simulink model "EMPCTower"  (R2021a)
settings: Solver=FixedStepDiscrete  StartTime=0.0  StopTime=120  FixedStep=Parameters.Ts  RelTol=1e-3
values from neighbouring files (symbols this model uses):
  Parameters =     [Parameters.mat]
undefined symbols (not defined in the file or in its folder): DeriveCp, DeriveFT, DriveTrain, EMPCController_Tower, TowerDynamic
settings Model: Creator=zfeng1  LastModifiedBy=zfeng1

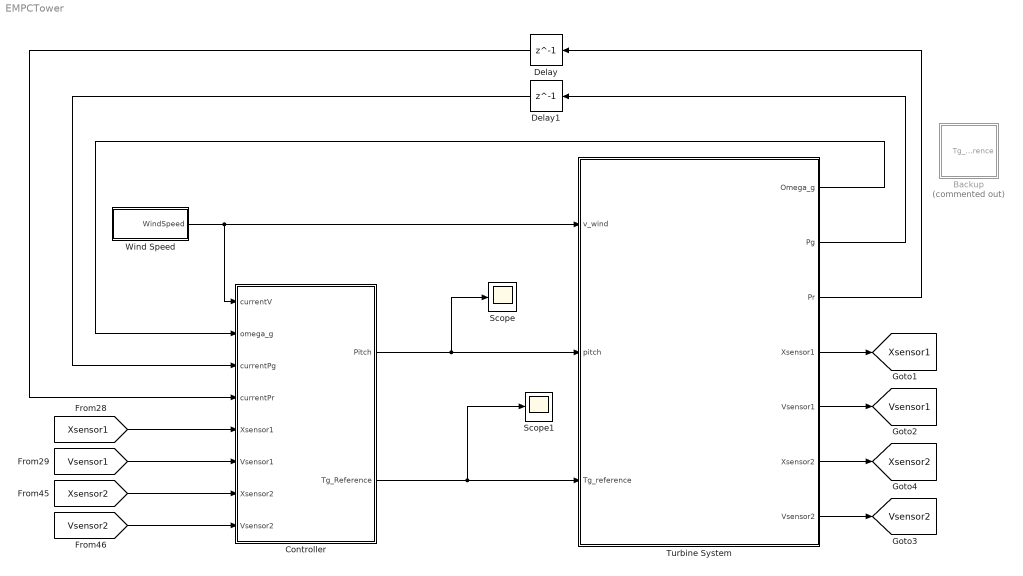
== system EMPCTower ==
  Backup : Subsystem  Commented=on
  Controller : Subsystem
  Delay : Delay  DelayLength=1  InitialCondition=0
  Delay1 : Delay  DelayLength=1  InitialCondition=0
  Scope : Scope
  Scope1 : Scope
  Turbine System : Subsystem
  Wind Speed : Subsystem
  tag scope: Vsensor1=global, Vsensor2=global, Xsensor1=global, Xsensor2=global
  wires:
  [Vsensor1] -> Controller/6(Vsensor1)
  [Vsensor2] -> Controller/8(Vsensor2)
  [Xsensor2] -> Controller/7(Xsensor2)
  [Xsensor1] -> Controller/5(Xsensor1)
  Wind Speed/1(WindSpeed) -> Controller/1(currentV), Turbine System/1(v_wind)
  Controller/1(Pitch) -> Scope/1, Turbine System/2(pitch)
  Controller/2(Tg_Reference) -> Scope1/1, Turbine System/3(Tg_reference)
  Turbine System/4(Xsensor1) -> [Xsensor1]
  Turbine System/5(Vsensor1) -> [Vsensor1]
  Turbine System/6(Xsensor2) -> [Xsensor2]
  Turbine System/7(Vsensor2) -> [Vsensor2]
  Turbine System/3(Pr) -> Delay/1
  Delay/1 -> Controller/4(currentPr)
  Turbine System/2(Pg) -> Delay1/1
  Delay1/1 -> Controller/3(currentPg)
  Turbine System/1(Omega_g) -> Controller/2(omega_g)

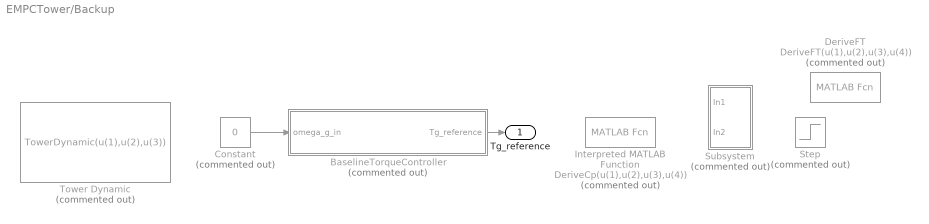
== system EMPCTower/Backup ==
  BaselineTorqueController : MATLAB Function  Commented=on  TreatAsAtomicUnit=on
  Constant : Constant  Commented=on  Value=0
  DeriveFT : MATLABFcn  Commented=on  MATLABFcn=DeriveFT(u(1),u(2),u(3),u(4))
  Interpreted MATLAB Function : MATLABFcn  Commented=on  MATLABFcn=DeriveCp(u(1),u(2),u(3),u(4))
  Step : Step  Commented=on  Time=200  Before=11  After=12  SampleTime=0
  Subsystem : Subsystem  Commented=on
  Tower Dynamic : MATLABFcn  Commented=on  MATLABFcn=TowerDynamic(u(1),u(2),u(3))
  Tg_reference : Outport
  wires:
  Constant/1 -> BaselineTorqueController/1(omega_g_in)
  BaselineTorqueController/1(Tg_reference) -> Tg_reference/1

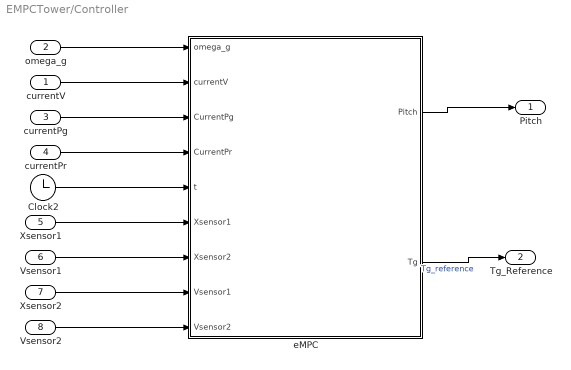
== system EMPCTower/Controller ==
  currentV : Inport
  omega_g : Inport  Port=2
  currentPg : Inport  Port=3
  currentPr : Inport  Port=4
  Xsensor1 : Inport  Port=5
  Vsensor1 : Inport  Port=6
  Xsensor2 : Inport  Port=7
  Vsensor2 : Inport  Port=8
  Clock2 : Clock
  eMPC : Subsystem
  Pitch : Outport
  Tg_Reference : Outport  Port=2
  wires:
  omega_g/1 -> eMPC/1(omega_g)
  currentV/1 -> eMPC/2(currentV)
  Clock2/1 -> eMPC/5(t)
  eMPC/1(Pitch) -> Pitch/1
  Xsensor1/1 -> eMPC/6(Xsensor1)
  Vsensor1/1 -> eMPC/7(Xsensor2)
  Xsensor2/1 -> eMPC/8(Vsensor1)
  Vsensor2/1 -> eMPC/9(Vsensor2)
  eMPC/2(Tg) -> Tg_Reference/1  "Tg_reference"
  currentPg/1 -> eMPC/3(CurrentPg)
  currentPr/1 -> eMPC/4(CurrentPr)

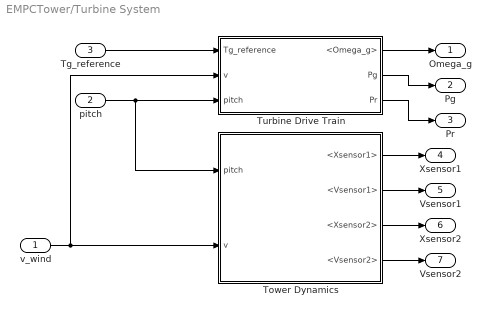
== system EMPCTower/Turbine System ==
  v_wind : Inport
  pitch : Inport  Port=2
  Tg_reference : Inport  Port=3
  Tower Dynamics : Subsystem
  Turbine Drive Train : Subsystem
  Omega_g : Outport
  Pg : Outport  Port=2
  Pr : Outport  Port=3
  Xsensor1 : Outport  Port=4
  Vsensor1 : Outport  Port=5
  Xsensor2 : Outport  Port=6
  Vsensor2 : Outport  Port=7
  wires:
  pitch/1 -> Turbine Drive Train/3(pitch), Tower Dynamics/1(pitch)
  v_wind/1 -> Turbine Drive Train/2(v), Tower Dynamics/2(v)
  Tg_reference/1 -> Turbine Drive Train/1(Tg_reference)
  Turbine Drive Train/1(<Omega_g>) -> Omega_g/1
  Tower Dynamics/1(<Xsensor1>) -> Xsensor1/1
  Tower Dynamics/2(<Vsensor1>) -> Vsensor1/1
  Tower Dynamics/3(<Xsensor2>) -> Xsensor2/1
  Tower Dynamics/4(<Vsensor2>) -> Vsensor2/1
  Turbine Drive Train/3(Pr) -> Pr/1
  Turbine Drive Train/2(Pg) -> Pg/1

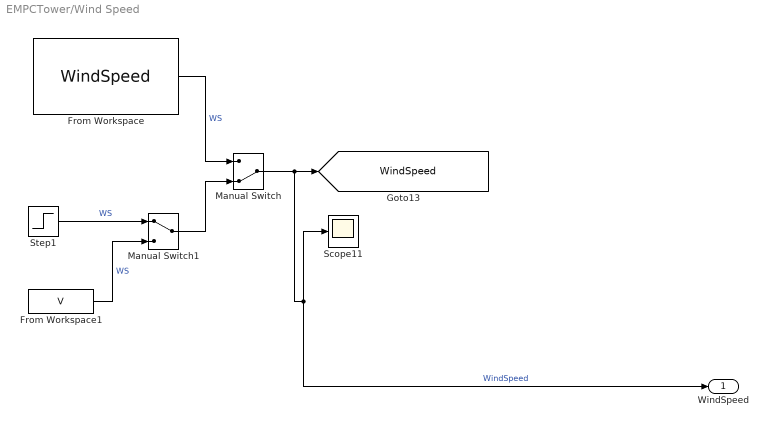
== system EMPCTower/Wind Speed ==
  From Workspace : FromWorkspace  VariableName=WindSpeed  SampleTime=Parameters.Ts
  From Workspace1 : FromWorkspace  VariableName=V
  Manual Switch : ManualSwitch  CurrentSetting=0
  Manual Switch1 : ManualSwitch
  Scope11 : Scope
  Step1 : Step  Time=0  Before=5  After=6  SampleTime=0
  WindSpeed : Outport
  tag scope: WindSpeed=global
  wires:
  Manual Switch1/1 -> Manual Switch/2
  Step1/1 -> Manual Switch1/1  "WS"
  Manual Switch/1 -> WindSpeed/1, Scope11/1, [WindSpeed]  "WindSpeed"
  From Workspace/1 -> Manual Switch/1  "WS"
  From Workspace1/1 -> Manual Switch1/2  "WS"

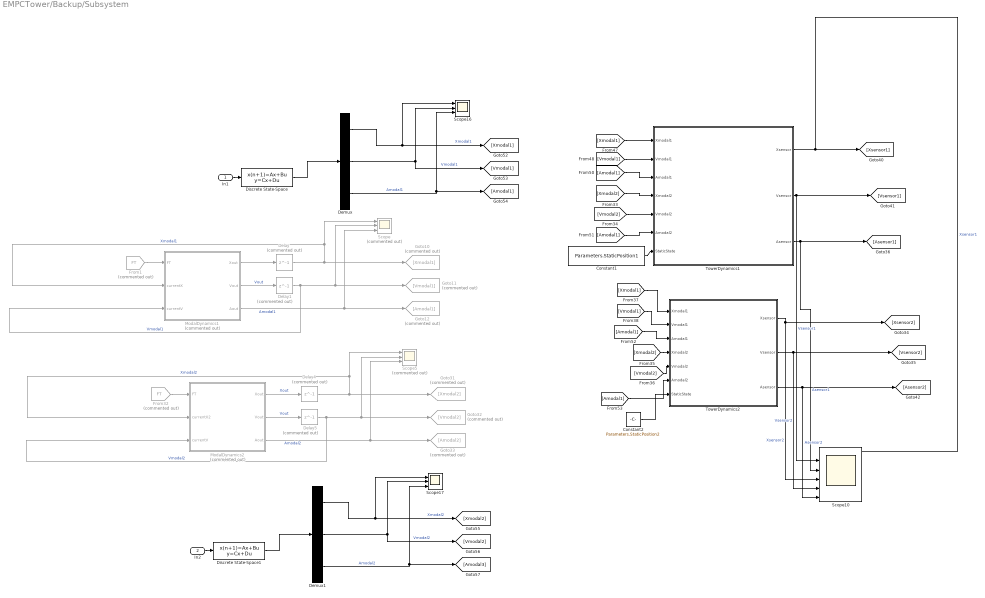
== system EMPCTower/Backup/Subsystem ==
  In1 : Inport
  In2 : Inport  Port=2
  Constant1 : Constant  Value=Parameters.StaticPosition1
  Constant2 : Constant  Value=Parameters.StaticPosition2
  Delay{,1,4..5} (4 alike) : Delay  Commented=on  DelayLength=1  InitialCondition=0  SampleTime=Parameters.Ts
  Demux : Demux  Outputs=3
  Demux1 : Demux  Outputs=3
  Discrete State-Space : DiscreteStateSpace  A=Parameters.sys_tower_fa_d.Am1  B=Parameters.sys_tower_fa_d.Bm1  C=Parameters.sys_tower_fa_d.Cm1  D=Parameters.sys_tower_fa_d.Dm1  SampleTime=-1
  Discrete State-Space1 : DiscreteStateSpace  A=Parameters.sys_tower_fa_d.Am2  B=Parameters.sys_tower_fa_d.Bm2  C=Parameters.sys_tower_fa_d.Cm2  D=Parameters.sys_tower_fa_d.Dm2  SampleTime=-1
  From1 : From  Commented=on  GotoTag=FT
  From32 : From  Commented=on  GotoTag=FT
  Goto10 : Goto  Commented=on  GotoTag=Xmodal1
  Goto11 : Goto  Commented=on  GotoTag=Vmodal1
  Goto12 : Goto  Commented=on  GotoTag=Amodal1
  Goto31 : Goto  Commented=on  GotoTag=Xmodal2
  Goto32 : Goto  Commented=on  GotoTag=Vmodal2
  Goto33 : Goto  Commented=on  GotoTag=Amodal2
  ModalDynamics1 : MATLAB Function  Commented=on  TreatAsAtomicUnit=on
  ModalDynamics2 : MATLAB Function  Commented=on  TreatAsAtomicUnit=on
  Scope : Scope  Commented=on  NumInputPorts=3
  Scope10 : Scope  NumInputPorts=6
  Scope16 : Scope  NumInputPorts=3
  Scope17 : Scope  NumInputPorts=3
  Scope5 : Scope  Commented=on  NumInputPorts=3
  TowerDynamics1 : MATLAB Function  TreatAsAtomicUnit=on
  TowerDynamics2 : MATLAB Function  TreatAsAtomicUnit=on
  wires:
  TowerDynamics1/2(Vsensor) -> [Vsensor1], Scope10/2  "Vsensor1"
  Demux/3 -> Scope16/3, [Amodal1]  "Amodal1"
  In1/1 -> Discrete State-Space/1
  ModalDynamics1/3(Aout) -> Scope/3, Goto12/1  "Amodal1"
  Delay4/1 -> ModalDynamics2/2(currentX2), Scope5/1, Goto31/1  "Xmodal2"
  In2/1 -> Discrete State-Space1/1
  Demux/2 -> Scope16/2, [Vmodal1]  "Vmodal1"
  Demux1/2 -> Scope17/2, [Vmodal2]  "Vmodal2"
  Discrete State-Space1/1 -> Demux1/1
  From1/1 -> ModalDynamics1/1(FT)
  Demux1/3 -> Scope17/3, [Amodal3]  "Amodal2"
  Demux/1 -> Scope16/1, [Xmodal1]  "Xmodal1"
  Discrete State-Space/1 -> Demux/1
  Constant1/1 -> TowerDynamics1/7(StaticState)
  [Vmodal1] -> TowerDynamics1/2(Vmodal1)
  ModalDynamics1/1(Xout) -> Delay/1
  TowerDynamics1/1(Xsensor) -> [Xsensor1], Scope10/1  "Xsensor1"
  [Amodal1] -> TowerDynamics2/6(Amodal2)
  [Amodal1] -> TowerDynamics1/6(Amodal2)
  ModalDynamics1/2(Vout) -> Delay1/1  "Vout"
  Delay/1 -> ModalDynamics1/2(currentX), Scope/1, Goto10/1  "Xmodal1"
  ModalDynamics2/3(Aout) -> Scope5/3, Goto33/1  "Amodal2"
  [Amodal1] -> TowerDynamics2/3(Amodal1)
  TowerDynamics2/3(Asensor) -> Scope10/6, [Asensor2]  "Asensor2"
  Constant2/1 -> TowerDynamics2/7(StaticState)
  Delay1/1 -> ModalDynamics1/3(currentV), Goto11/1, Scope/2  "Vmodal1"
  TowerDynamics1/3(Asensor) -> Scope10/3, [Asensor1]  "Asensor1"
  ModalDynamics2/2(Vout) -> Delay5/1  "Vout"
  [Xmodal2] -> TowerDynamics2/4(Xmodal2)
  [Vmodal2] -> TowerDynamics1/5(Vmodal2)
  [Xmodal1] -> TowerDynamics2/1(Xmodal1)
  ModalDynamics2/1(Xout) -> Delay4/1  "Xout"
  [Xmodal1] -> TowerDynamics1/1(Xmodal1)
  [Xmodal2] -> TowerDynamics1/4(Xmodal2)
  TowerDynamics2/2(Vsensor) -> Scope10/5, [Vsensor2]  "Vsensor2"
  From32/1 -> ModalDynamics2/1(FT)
  [Vmodal2] -> TowerDynamics2/5(Vmodal2)
  [Amodal1] -> TowerDynamics1/3(Amodal1)
  [Vmodal1] -> TowerDynamics2/2(Vmodal1)
  TowerDynamics2/1(Xsensor) -> Scope10/4, [Xsensor2]  "Xsensor2"
  Delay5/1 -> ModalDynamics2/3(currentV), Goto32/1, Scope5/2  "Vmodal2"
  Demux1/1 -> Scope17/1, [Xmodal2]  "Xmodal2"

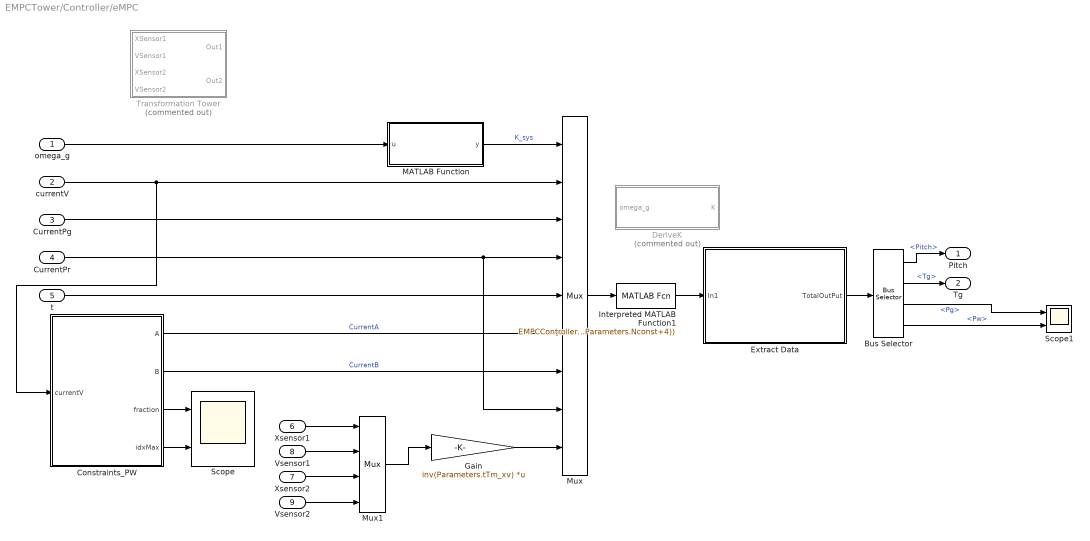
== system EMPCTower/Controller/eMPC ==
  omega_g : Inport
  currentV : Inport  Port=2
  CurrentPg : Inport  Port=3
  CurrentPr : Inport  Port=4
  t : Inport  Port=5
  Xsensor1 : Inport  Port=6
  Xsensor2 : Inport  Port=7
  Vsensor1 : Inport  Port=8
  Vsensor2 : Inport  Port=9
  Bus Selector : BusSelector  OutputSignals=Pitch,Tg,Pg,Pw
  Constraints_PW : MATLAB Function  TreatAsAtomicUnit=on  SystemSampleTime=Parameters.Ts
  DeriveK : MATLAB Function  Commented=on  TreatAsAtomicUnit=on  SystemSampleTime=Parameters.DT
  Extract Data : Subsystem
  Gain : Gain  Gain=inv(Parameters.tTm_xv)  Multiplication=Matrix(K*u) (u vector)
  Interpreted MATLAB Function1 : MATLABFcn  MATLABFcn=EMPCController_Tower(u(1),u(2),u(3),u(4),u(5),u(6:1:6+Parameters.Nconst-1),u(6+Parameters.Nconst:1:6+2*Parameters.Nconst-1),u(6+2*Parameters.Nconst),u(6+2*Parameters.Nconst+1:6+2*Parameters.Nconst+2),u(6+2*Parameters.Nconst+3:6+2*Parameters.Nconst+4))
  MATLAB Function : MATLAB Function  TreatAsAtomicUnit=on
  Mux : Mux  Inputs=9
  Mux1 : Mux
  Scope : Scope  NumInputPorts=2
  Scope1 : Scope  NumInputPorts=2
  Transformation Tower : Subsystem  Commented=on
  Pitch : Outport
  Tg : Outport  Port=2
  wires:
  Constraints_PW/1(A) -> Mux/6  "CurrentA"
  currentV/1 -> Mux/2, Constraints_PW/1(currentV)
  Mux/1 -> Interpreted MATLAB Function1/1
  MATLAB Function/1(y) -> Mux/1  "K_sys"
  Constraints_PW/2(B) -> Mux/7  "CurrentB"
  omega_g/1 -> MATLAB Function/1(u)
  t/1 -> Mux/5
  Constraints_PW/3(fraction) -> Scope/1
  Constraints_PW/4(idxMax) -> Scope/2
  Interpreted MATLAB Function1/1 -> Extract Data/1(In1)
  Xsensor1/1 -> Mux1/1
  Vsensor1/1 -> Mux1/2
  Xsensor2/1 -> Mux1/3
  Vsensor2/1 -> Mux1/4
  Mux1/1 -> Gain/1
  Extract Data/1(TotalOutPut) -> Bus Selector/1
  Bus Selector/1 -> Pitch/1  "<Pitch>"
  Bus Selector/2 -> Tg/1  "<Tg>"
  Bus Selector/3 -> Scope1/1  "<Pg>"
  Bus Selector/4 -> Scope1/2  "<Pw>"
  Gain/1 -> Mux/9
  CurrentPg/1 -> Mux/3
  CurrentPr/1 -> Mux/8, Mux/4

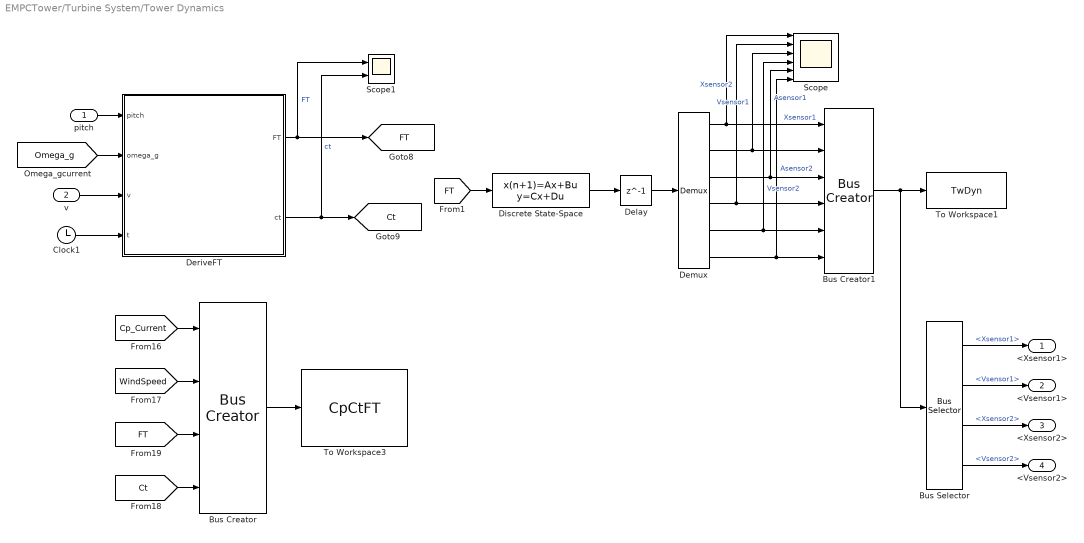
== system EMPCTower/Turbine System/Tower Dynamics ==
  pitch : Inport
  v : Inport  Port=2
  " DeriveFT" : MATLAB Function  TreatAsAtomicUnit=on
  Bus Creator : BusCreator  Inputs=4
  Bus Creator1 : BusCreator  Inputs=6
  Bus Selector : BusSelector  OutputSignals=Xsensor1,Vsensor1,Xsensor2,Vsensor2
  Clock1 : Clock
  Delay : Delay  DelayLength=1  InitialCondition=0
  Demux : Demux  Outputs=6
  Discrete State-Space : DiscreteStateSpace  A=Parameters.sys_tower_fa_d.A  B=Parameters.sys_tower_fa_d.B  C=Parameters.sys_tower_fa_d.C  D=Parameters.sys_tower_fa_d.D  SampleTime=Parameters.Ts
  Scope : Scope  NumInputPorts=6
  Scope1 : Scope  NumInputPorts=2
  To Workspace1 : ToWorkspace  VariableName=TwDyn  SaveFormat=Timeseries  SampleTime=-1
  To Workspace3 : ToWorkspace  VariableName=CpCtFT  SaveFormat=Timeseries  SampleTime=-1
  <Xsensor1> : Outport
  <Vsensor1> : Outport  Port=2
  <Xsensor2> : Outport  Port=3
  <Vsensor2> : Outport  Port=4
  tag scope: Ct=global, FT=global
  wires:
  [FT] -> Discrete State-Space/1
  Clock1/1 -> " DeriveFT"/4(t)
  Bus Creator1/1 -> Bus Selector/1, To Workspace1/1
  Demux/5 -> Bus Creator1/5, Scope/4  "Vsensor2"
  Demux/3 -> Scope/5, Bus Creator1/3  "Asensor1"
  pitch/1 -> " DeriveFT"/1(pitch)
  Demux/6 -> Bus Creator1/6, Scope/6  "Asensor2"
  Demux/2 -> Scope/3, Bus Creator1/2  "Vsensor1"
  Demux/4 -> Bus Creator1/4, Scope/2  "Xsensor2"
  " DeriveFT"/2(ct) -> [Ct], Scope1/2  "ct"
  " DeriveFT"/1(FT) -> [FT], Scope1/1  "FT"
  Demux/1 -> Scope/1, Bus Creator1/1  "Xsensor1"
  Bus Selector/1 -> <Xsensor1>/1  "<Xsensor1>"
  [Omega_g] -> " DeriveFT"/2(omega_g)
  Bus Selector/4 -> <Vsensor2>/1  "<Vsensor2>"
  Discrete State-Space/1 -> Delay/1
  Bus Selector/2 -> <Vsensor1>/1  "<Vsensor1>"
  v/1 -> " DeriveFT"/3(v)
  Bus Selector/3 -> <Xsensor2>/1  "<Xsensor2>"
  Bus Creator/1 -> To Workspace3/1
  [WindSpeed] -> Bus Creator/2
  [Ct] -> Bus Creator/4
  [Cp_Current] -> Bus Creator/1
  [FT] -> Bus Creator/3
  Delay/1 -> Demux/1

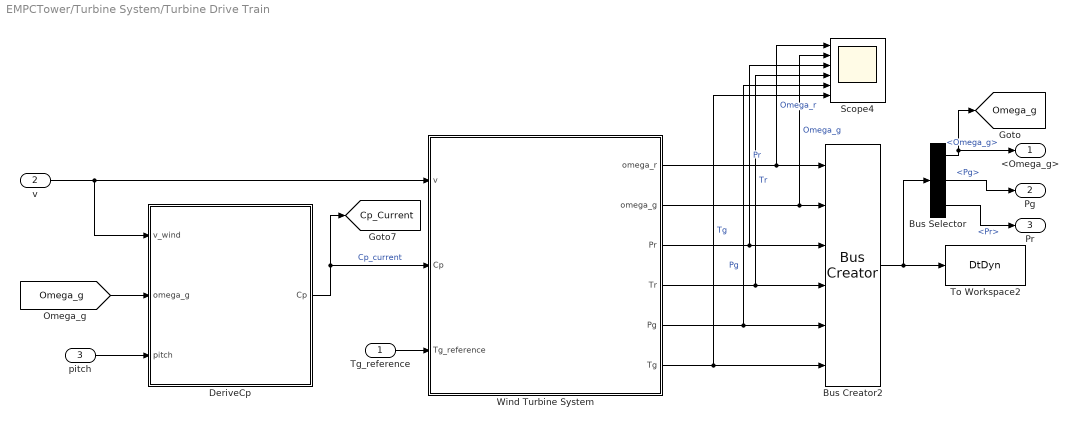
== system EMPCTower/Turbine System/Turbine Drive Train ==
  Tg_reference : Inport
  v : Inport  Port=2
  pitch : Inport  Port=3
  Bus Creator2 : BusCreator  Inputs=6
  Bus Selector : BusSelector  OutputSignals=Omega_g,Pg,Pr
  DeriveCp : MATLAB Function  TreatAsAtomicUnit=on
  Scope4 : Scope  NumInputPorts=6
  To Workspace2 : ToWorkspace  VariableName=DtDyn  SaveFormat=Timeseries  SampleTime=-1
  Wind Turbine System : Subsystem
  <Omega_g> : Outport
  Pg : Outport  Port=2
  Pr : Outport  Port=3
  tag scope: Cp_Current=global, Omega_g=global
  wires:
  Wind Turbine System/4(Tr) -> Scope4/4, Bus Creator2/4  "Tr"
  Wind Turbine System/5(Pg) -> Scope4/5, Bus Creator2/5  "Pg"
  v/1 -> DeriveCp/1(v_wind), Wind Turbine System/1(v)
  Wind Turbine System/6(Tg) -> Scope4/6, Bus Creator2/6  "Tg"
  Wind Turbine System/2(omega_g) -> Scope4/2, Bus Creator2/2  "Omega_g"
  Wind Turbine System/1(omega_r) -> Scope4/1, Bus Creator2/1  "Omega_r"
  DeriveCp/1(Cp) -> Wind Turbine System/2(Cp), [Cp_Current]  "Cp_current"
  Wind Turbine System/3(Pr) -> Scope4/3, Bus Creator2/3  "Pr"
  [Omega_g] -> DeriveCp/2(omega_g)
  Bus Creator2/1 -> Bus Selector/1, To Workspace2/1
  Tg_reference/1 -> Wind Turbine System/3(Tg_reference)
  pitch/1 -> DeriveCp/3(pitch)
  Bus Selector/1 -> <Omega_g>/1, [Omega_g]  "<Omega_g>"
  Bus Selector/3 -> Pr/1  "<Pr>"
  Bus Selector/2 -> Pg/1  "<Pg>"

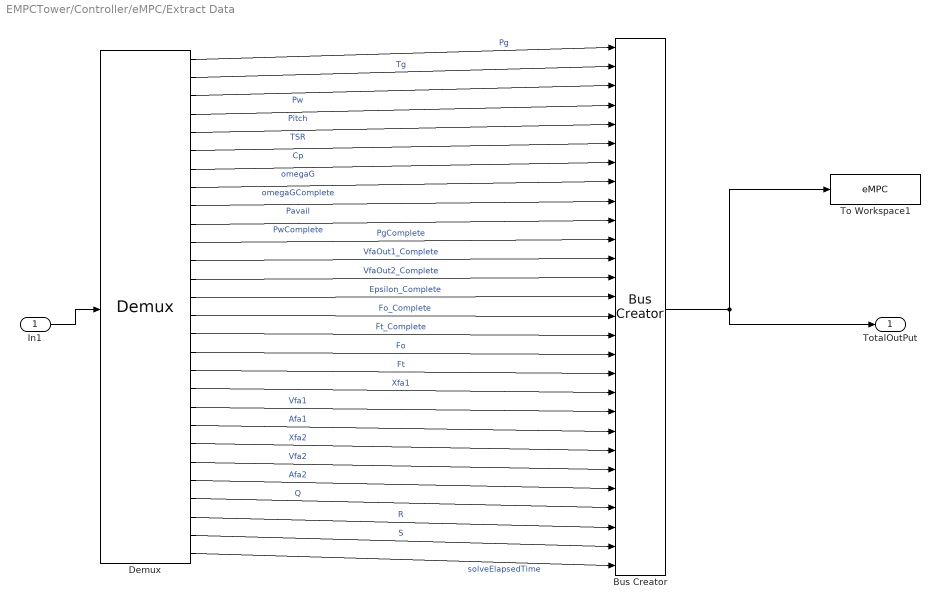
== system EMPCTower/Controller/eMPC/Extract Data ==
  In1 : Inport
  Bus Creator : BusCreator  Inputs=28
  Demux : Demux  Outputs=[1 1 1 1 1 1 1 Parameters.Np Parameters.Np+1 Parameters.Np+1 Parameters.Np+1 Parameters.Np Parameters.Np Parameters.Np Parameters.Np Parameters.Np 1 1 1 1 1 1 1 1 1 1 1 -1]
      settings: DisplayOption=none
  To Workspace1 : ToWorkspace  VariableName=eMPC  SaveFormat=Timeseries  SampleTime=-1
  TotalOutPut : Outport
  wires:
  Demux/9 -> Bus Creator/9  "Pavail"
  Demux/4 -> Bus Creator/4  "Pitch"
  Demux/5 -> Bus Creator/5  "TSR"
  Demux/1 -> Bus Creator/1  "Pg"
  Demux/10 -> Bus Creator/10  "PwComplete"
  Demux/27 -> Bus Creator/27  "S"
  Demux/2 -> Bus Creator/2  "Tg"
  Demux/25 -> Bus Creator/25  "Q"
  Demux/16 -> Bus Creator/16  "Ft_Complete"
  Demux/20 -> Bus Creator/20  "Vfa1"
  Demux/21 -> Bus Creator/21  "Afa1"
  Demux/14 -> Bus Creator/14  "Epsilon_Complete"
  Demux/24 -> Bus Creator/24  "Afa2"
  Demux/26 -> Bus Creator/26  "R"
  Demux/8 -> Bus Creator/8  "omegaGComplete"
  Bus Creator/1 -> TotalOutPut/1, To Workspace1/1
  Demux/17 -> Bus Creator/17  "Fo"
  Demux/22 -> Bus Creator/22  "Xfa2"
  Demux/15 -> Bus Creator/15  "Fo_Complete"
  Demux/19 -> Bus Creator/19  "Xfa1"
  In1/1 -> Demux/1
  Demux/12 -> Bus Creator/12  "VfaOut1_Complete"
  Demux/6 -> Bus Creator/6  "Cp"
  Demux/18 -> Bus Creator/18  "Ft"
  Demux/28 -> Bus Creator/28  "solveElapsedTime"
  Demux/11 -> Bus Creator/11  "PgComplete"
  Demux/3 -> Bus Creator/3  "Pw"
  Demux/23 -> Bus Creator/23  "Vfa2"
  Demux/13 -> Bus Creator/13  "VfaOut2_Complete"
  Demux/7 -> Bus Creator/7  "omegaG"

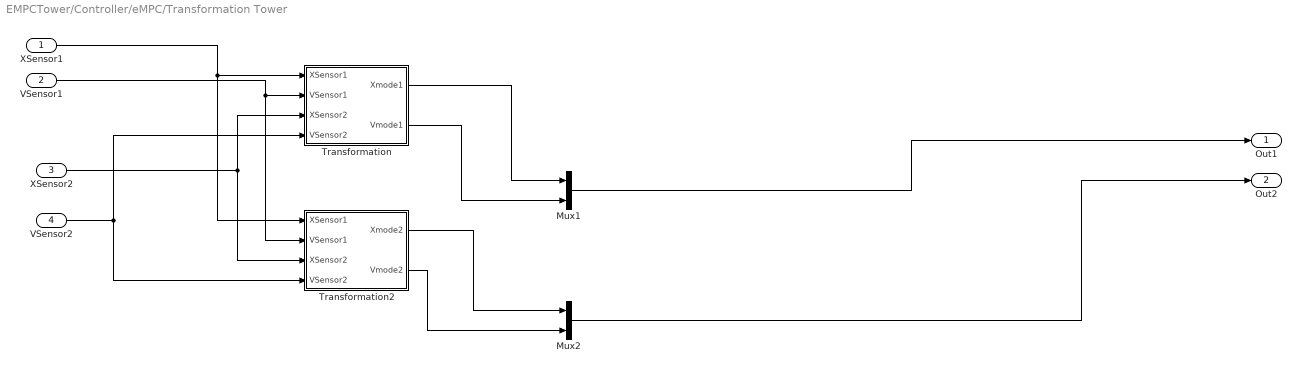
== system EMPCTower/Controller/eMPC/Transformation Tower ==
  XSensor1 : Inport
  VSensor1 : Inport  Port=2
  XSensor2 : Inport  Port=3
  VSensor2 : Inport  Port=4
  Mux1 : Mux  Inputs=2
  Mux2 : Mux  Inputs=2
  Transformation : MATLAB Function  TreatAsAtomicUnit=on
  Transformation2 : MATLAB Function  TreatAsAtomicUnit=on
  Out1 : Outport
  Out2 : Outport  Port=2
  wires:
  Transformation2/1(Xmode2) -> Mux2/1
  Mux1/1 -> Out1/1
  VSensor1/1 -> Transformation2/2(VSensor1), Transformation/2(VSensor1)
  VSensor2/1 -> Transformation2/4(VSensor2), Transformation/4(VSensor2)
  Transformation2/2(Vmode2) -> Mux2/2
  Transformation/2(Vmode1) -> Mux1/2
  XSensor1/1 -> Transformation2/1(XSensor1), Transformation/1(XSensor1)
  Transformation/1(Xmode1) -> Mux1/1
  XSensor2/1 -> Transformation2/3(XSensor2), Transformation/3(XSensor2)
  Mux2/1 -> Out2/1

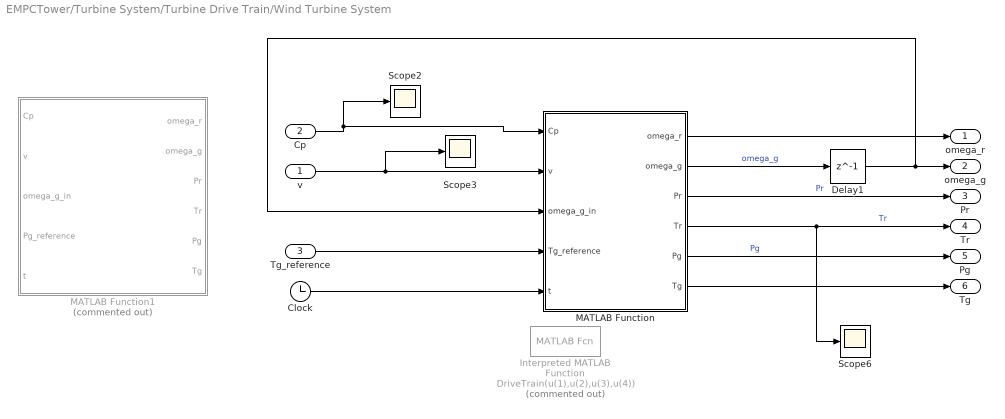
== system EMPCTower/Turbine System/Turbine Drive Train/Wind Turbine System ==
  v : Inport
  Cp : Inport  Port=2
  Tg_reference : Inport  Port=3
  Clock : Clock
  Delay1 : Delay  DelayLength=1  InitialCondition=50  SampleTime=Parameters.Ts
  Interpreted MATLAB Function : MATLABFcn  Commented=on  MATLABFcn=DriveTrain(u(1),u(2),u(3),u(4))
  MATLAB Function : MATLAB Function  TreatAsAtomicUnit=on
  MATLAB Function1 : MATLAB Function  Commented=on  TreatAsAtomicUnit=on
  Scope2 : Scope
  Scope3 : Scope
  Scope6 : Scope
  omega_r : Outport
  omega_g : Outport  Port=2
  Pr : Outport  Port=3
  Tr : Outport  Port=4
  Pg : Outport  Port=5
  Tg : Outport  Port=6
  wires:
  v/1 -> MATLAB Function/2(v), Scope3/1
  MATLAB Function/4(Tr) -> Tr/1, Scope6/1  "Tr"
  Cp/1 -> MATLAB Function/1(Cp), Scope2/1
  MATLAB Function/2(omega_g) -> Delay1/1  "omega_g"
  Clock/1 -> MATLAB Function/5(t)
  Delay1/1 -> MATLAB Function/3(omega_g_in), omega_g/1
  MATLAB Function/6(Tg) -> Tg/1
  Tg_reference/1 -> MATLAB Function/4(Tg_reference)
  MATLAB Function/3(Pr) -> Pr/1  "Pr"
  MATLAB Function/5(Pg) -> Pg/1  "Pg"
  MATLAB Function/1(omega_r) -> omega_r/1

== matlab function EMPCTower/Turbine System/Turbine Drive Train/Wind Turbine System/MATLAB Function1 ==
  data: Cp input; omega_r output; v input; omega_g_in input; Pg_reference input; t input; omega_g output; Pr output; Tr output; Pg output; Tg output; Parameters parameter
function [omega_r, omega_g, Pr, Tr, Pg, Tg] = fcn(Cp,v, omega_g_in, Pg_reference,t,Parameters)

if t == 0
    omega_g_in = 41.6471;
end
    
    omega_r_in = omega_g_in/Parameters.G;

%     Tg = 2.3323*omega_g_in^2;
    %Tg = Tg_reference;
    Pr = 1/2*Parameters.rho*pi*Parameters.R^2*Cp*v^3;
    Tr = Pr/omega_r_in;
    Pg = Pg_reference;
    
    K_current = 1/2*Parameters.Je*omega_g_in^2;
    K_current_scaled = K_current/Parameters.ScaleK;
    Delta_K_scaled = (Pr-Pg/Parameters.Effic)/Parameters.ScaleK*Parameters.Ts;
    K_out_scaled = K_current_scaled+Delta_K_scaled;
    K_out = K_out_scaled*Parameters.ScaleK;
%     K_out = (K_current/Parameters.ScaleK+ (Pr-Pg_reference/Parameters.Effic)/Parameters.ScaleP*Parameters.Ts)*Parameters.ScaleK;
    
    omega_g = sqrt(K_out*2/Parameters.Je);
    Tg = Pg/Parameters.Effic/omega_g;
    
%     omega_g = Parameters.Ts*(Tr/Parameters.G-Tg)/Parameters.Je+omega_g_in;
    omega_r = omega_g/Parameters.G;

%     Pg = Tg*omega_g;

    WTout = [omega_r;omega_g;Pr;Tr;Pg;Tg];

== matlab function EMPCTower/Backup/Subsystem/ModalDynamics1 ==
  data: FT input; currentX input; currentV input; Parameters parameter; Xout output; Vout output; Aout output
function [Xout,Vout,Aout]=fcn(FT,currentX, currentV,Parameters)

towerstates = Parameters.sys_tower_fa_d.Am1*[currentX;currentV]+ Parameters.sys_tower_fa_d.Bm1*FT;
towerout = Parameters.sys_tower_fa_d.Cm1*[currentX;currentV]+ Parameters.sys_tower_fa_d.Dm1*FT;
Xout =towerstates(1);
Vout = towerstates(2);
Aout = towerout(3);

== matlab function EMPCTower/Backup/Subsystem/TowerDynamics2 ==
  data: Xmodal1 input; Vmodal1 input; Amodal1 input; Xmodal2 input; Xsensor output; Vsensor output; Vmodal2 input; Amodal2 input; StaticState input; Asensor output
function [Xsensor,Vsensor,Asensor]=fcn(Xmodal1,Vmodal1,Amodal1,Xmodal2,Vmodal2,Amodal2,StaticState)

Xsensor = Xmodal1*StaticState(1) + Xmodal2*StaticState(2);
Vsensor = Vmodal1*StaticState(1)+ Vmodal2*StaticState(2);
Asensor = Amodal1*StaticState(1)+ Amodal2*StaticState(2);

== matlab function EMPCTower/Controller/eMPC/Transformation Tower/Transformation ==
  data: XSensor1 input; VSensor1 input; XSensor2 input; VSensor2 input; Xmode1 output; Parameters parameter; Vmode1 output
function [Xmode1,Vmode1] = fcn(XSensor1,VSensor1,XSensor2,VSensor2,Parameters)

Xmode1 = (Parameters.Tmatrix(2,2)*XSensor1 - Parameters.Tmatrix(1,2) * XSensor2)...
         /(Parameters.Tmatrix(1,1) *Parameters.Tmatrix(2,2) -Parameters.Tmatrix(2,1) *Parameters.Tmatrix(2,2) );
Vmode1 = (Parameters.Tmatrix(2,2) *VSensor1- Parameters.Tmatrix(1,2) * VSensor2)...
         /(Parameters.Tmatrix(1,1) *Parameters.Tmatrix(2,2) -Parameters.Tmatrix(2,1) *Parameters.Tmatrix(1,2) );

== matlab function EMPCTower/Controller/eMPC/Transformation Tower/Transformation2 ==
  data: XSensor1 input; VSensor1 input; XSensor2 input; VSensor2 input; Xmode2 output; Parameters parameter; Vmode2 output
function [Xmode2,Vmode2] = fcn( XSensor1,VSensor1, XSensor2,VSensor2,Parameters)

Xmode2 = -(Parameters.Tmatrix(2,1) * XSensor1 - Parameters.Tmatrix(1,1)  * XSensor2)...
         /(Parameters.Tmatrix(1,1) *Parameters.Tmatrix(2,2) -Parameters.Tmatrix(2,1)*Parameters.Tmatrix(1,2));
Vmode2 = (Parameters.Tmatrix(2,1)* VSensor1 - Parameters.Tmatrix(1,1)  * VSensor2)...
         /(Parameters.Tmatrix(2,1) *Parameters.Tmatrix(1,2) -Parameters.Tmatrix(2,2) *Parameters.Tmatrix(1,1) );

== matlab function EMPCTower/Backup/Subsystem/TowerDynamics1 ==
  data: Xmodal1 input; Vmodal1 input; Amodal1 input; Xmodal2 input; Xsensor output; Vsensor output; Vmodal2 input; Amodal2 input; StaticState input; Asensor output
function [Xsensor,Vsensor,Asensor]=fcn(Xmodal1,Vmodal1,Amodal1,Xmodal2,Vmodal2,Amodal2,StaticState)

Xsensor = Xmodal1*StaticState(1) + Xmodal2*StaticState(2);
Vsensor = Vmodal1*StaticState(1)+ Vmodal2*StaticState(2);
Asensor = Amodal1*StaticState(1)+ Amodal2*StaticState(2);

== matlab function EMPCTower/Turbine System/Turbine Drive Train/DeriveCp ==
  settings: sampleTime=Ts
  data: v_wind input; Cp output; omega_g input; pitch input; Parameters parameter
function Cp = fcn(v_wind, omega_g, pitch, Parameters)

%     if t == 0
%         v_wind = 6;
%         omega_g = 41.6471;
%     end
    
    omega_r = omega_g/Parameters.G;
    
    TSR=omega_r*Parameters.R/v_wind;
    
%     if TSR < 2
%         TSR = max(2,TSR);
%         Cp_derived = max(interp2(Tables.TSR,Tables.Pitch,Tables.Cp,TSR,pitch,'spline'),0);
%     else
%         TSR = max(2,min(10,TSR));
%         Cp_derived = max(interp2(Tables.TSR,Tables.Pitch,Tables.Cp,TSR,pitch,'spline'),0);
%     end
Cp_derived = max(interp2(Parameters.Rotor_Lamda,Parameters.Rotor_Pitch,Parameters.Rotor_cP,TSR,pitch,'spline'),0);
    
    Cp = Cp_derived;

== matlab function EMPCTower/Turbine System/Turbine Drive Train/Wind Turbine System/MATLAB Function ==
  settings: updateMethod=DISCRETE  sampleTime=Parameters.Ts
  data: Cp input; v input; omega_g_in input; Tg_reference input; omega_r output; t input; omega_g output; Pr output; Tr output; Pg output; Tg output; Parameters parameter
function [omega_r, omega_g, Pr, Tr, Pg, Tg] = fcn(Cp,v, omega_g_in, Tg_reference,t,Parameters)

% if t == 0
%     omega_g_in = 41.6471;
% end
    
    omega_r_in = omega_g_in/Parameters.G;
    Tg = Tg_reference;
    Pr = 1/2*Parameters.rho*pi*Parameters.R^2*Cp*v^3;
    Tr = Pr/omega_r_in;
    Delta_omega_g = Parameters.Ts*(Tr/Parameters.G-Tg/Parameters.Effic)/Parameters.Je;
    omega_g =omega_g_in + Delta_omega_g;
    omega_r = omega_g/Parameters.G;
    Pg = Tg*omega_g;

% 
% %     Tg = 2.3323*omega_g_in^2;
%     Tg = Tg_reference;
%     Pr = 1/2*Parameters.rho*pi*Parameters.R^2*Cp*v^3;
%     Tr = Pr/omega_r_in;
%     
%     omega_g = Parameters.Ts*(Tr/Parameters.G-Tg)/Parameters.Je+omega_g_in;
%     omega_r = omega_g/Parameters.G;
% 
%     Pg = Tg*omega_g;

    WTout = [omega_r;omega_g;Pr;Tr;Pg;Tg];

== matlab function EMPCTower/Turbine System/Tower Dynamics/ DeriveFT ==
  settings: sampleTime=Ts
  data: pitch input; FT output; omega_g input; v input; t input; Parameters parameter; ct output
function  [FT, ct]= fcn(pitch,omega_g,v,t, Parameters)


omega_r = omega_g/Parameters.G;
TSR = omega_r*Parameters.R/v;

% if TSR <2 
%     ct = 0;
% % else
%     TSR = max(2,min(10,TSR));
    ct = interp2(Parameters.Rotor_Lamda,Parameters.Rotor_Pitch,Parameters.Rotor_cT,TSR,pitch,'spline');
% end

FT = 1/2*Parameters.rho*pi*Parameters.R^2*ct*v^2;

== matlab function EMPCTower/Backup/Subsystem/ModalDynamics2 ==
  data: FT input; currentX2 input; currentV input; Parameters parameter; Xout output; Vout output; Aout output
function [Xout,Vout,Aout]=fcn(FT,currentX2, currentV,Parameters)

towerstates = Parameters.sys_tower_fa_d.Am2*[currentX2;currentV]+ Parameters.sys_tower_fa_d.Bm2*FT;
towerout = Parameters.sys_tower_fa_d.Cm2*[currentX2;currentV]+ Parameters.sys_tower_fa_d.Dm2*FT;
Xout = towerstates(1);
Vout = towerstates(2);
Aout = towerout(3);

== matlab function EMPCTower/Backup/BaselineTorqueController ==
  data: omega_g_in input; Tg_reference output
function Tg_reference = fcn(omega_g_in)

Tg_reference = 2.3323*omega_g_in^2;

== matlab function EMPCTower/Controller/eMPC/DeriveK ==
  settings: updateMethod=DISCRETE  sampleTime=Ts
  data: omega_g input; K output; Parameters parameter
function K = fcn(omega_g, Parameters)

K = 1/2*Parameters.J*omega_g^2;

== matlab function EMPCTower/Controller/eMPC/Constraints_PW ==
  settings: sampleTime=Ts
  data: currentV input size=1; A output size=[Parameters.Nconst,1]; B output size=[Parameters.Nconst,1]; Parameters parameter; fraction output; idxMax output
function [A,B, fraction, idxMax]  = fcn(currentV, Parameters)

% Prevent the wind speed fall outside 2-25 m/s range where the PWL
% functions are defined
currentV=max(min(currentV,25),2);

% Preallocation
A=zeros(Parameters.Nconst,1);
B=zeros(Parameters.Nconst,1);

% Determine the fraction for PWL function coefficient calculation
[~,idxMax]=max( ( (Parameters.BOUNDPW.V-currentV) >=0 ) * -50 + (Parameters.BOUNDPW.V-currentV) );
fraction=1-(currentV-Parameters.BOUNDPW.V(idxMax))/(Parameters.BOUNDPW.V(idxMax+1)-Parameters.BOUNDPW.V(idxMax));

% Calculate the PWL function coefficients
A=(Parameters.BOUNDPW.Ac(:,idxMax)*fraction+Parameters.BOUNDPW.Ac(:,idxMax+1)*(1-fraction));
B=(Parameters.BOUNDPW.Bc(:,idxMax)*fraction+Parameters.BOUNDPW.Bc(:,idxMax+1)*(1-fraction));

== matlab function EMPCTower/Controller/eMPC/MATLAB Function ==
  data: u input; y output; Parameters parameter
function y = fcn(u,Parameters)

y = 1/2*Parameters.Je*u^2;
